simulink model "exp_7"  (R2020a)
settings: Solver=VariableStepAuto  StartTime=0.0  StopTime=10.0  RelTol=1e-3
settings Model: Creator=hp  LastModifiedBy=hp

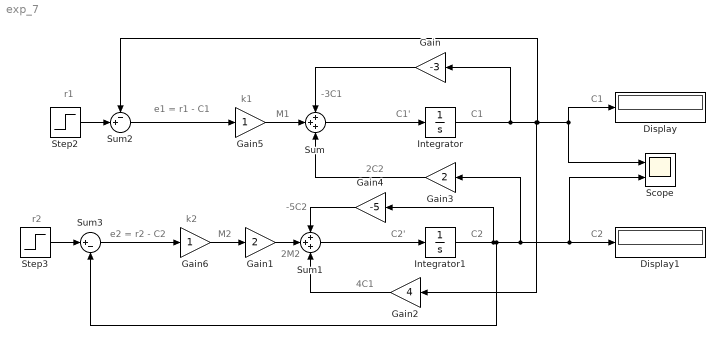
== system exp_7 ==
  note: C2
  note: -5C2
  note: 2M2
  note: -3C1
  note: M1
  note: C1
  note: 4C1
  note: C2
  note: C1
  note: C2'
  note: C1'
  note: 2C2
  note: M2
  note: r1
  note: r2
  note: e1 = r1 - C1
  note: e2 = r2 - C2
  note: k1
  note: k2
  Display : Display
  Display1 : Display
  Gain : Gain  Gain=-3
  Gain1 : Gain  Gain=2
  Gain2 : Gain  Gain=4
  Gain3 : Gain  Gain=2
  Gain4 : Gain  Gain=-5
  Gain5 : Gain
  Gain6 : Gain
  Integrator : Integrator
  Integrator1 : Integrator
  Scope : Scope  NumInputPorts=2
  Step2 : Step  Time=0  SampleTime=0
  Step3 : Step  Time=0  SampleTime=0
  Sum : Sum  Inputs=+++
  Sum1 : Sum  Inputs=+++
  Sum2 : Sum  Inputs=-+|
  Sum3 : Sum  Inputs=|+-
  wires:
  Sum/1 -> Integrator/1
  Gain6/1 -> Gain1/1
  Gain/1 -> Sum/1
  Gain5/1 -> Sum/2
  Integrator1/1 -> Gain4/1, Gain3/1, Scope/2, Display1/1, Sum3/2
  Sum1/1 -> Integrator1/1
  Gain2/1 -> Sum1/3
  Gain3/1 -> Sum/3
  Gain1/1 -> Sum1/2
  Gain4/1 -> Sum1/1
  Integrator/1 -> Sum2/1, Display/1, Scope/1, Gain2/1, Gain/1
  Sum2/1 -> Gain5/1
  Sum3/1 -> Gain6/1
  Step2/1 -> Sum2/2
  Step3/1 -> Sum3/1
